simulink model "try_nelin2"  (R2014b)
settings: Solver=ode45  StartTime=0.0  StopTime=10.0  RelTol=1e-3
values from neighbouring files (symbols this model uses):
  d = 39.73e-3    (= 0.03973)    [liniarizare_crazyflie.m]
  g = 9.81    [liniarizare_crazyflie.m]
  Ixx = 1.395e-05    [liniarizare_crazyflie.m]
  Iyy = 1.436e-05    [liniarizare_crazyflie.m]
  Izz = 2.173e-05    [liniarizare_crazyflie.m]
  m = 0.27    [liniarizare_crazyflie.m]
  Th_coef = 3.1582e-10    [liniarizare_crazyflie.m]
  To_coef = 7.9379e-12    [liniarizare_crazyflie.m]
settings Model: Creator=uidd7441  LastModifiedBy=uidd7441

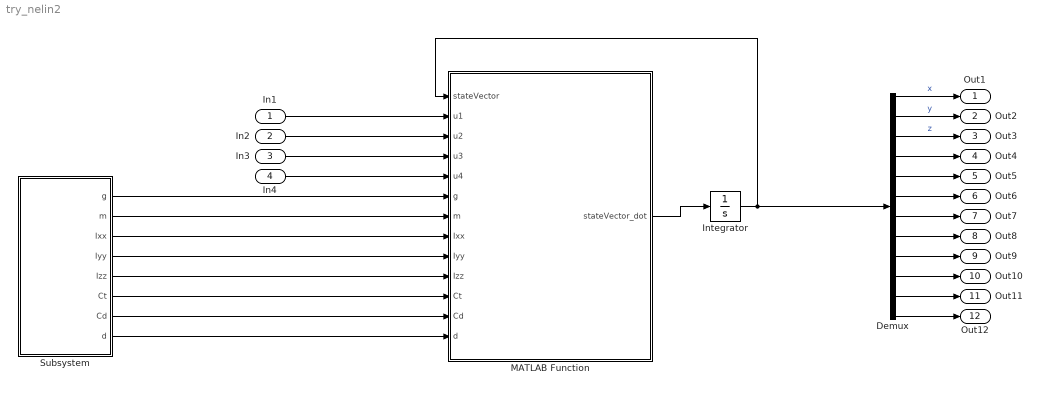
== system try_nelin2 ==
  In1 : Inport
  In2 : Inport  Port=2
  In3 : Inport  Port=3
  In4 : Inport  Port=4
  Demux : Demux  Outputs=12
  Integrator : Integrator  InitialCondition=[0 0 0 1 0 0 0 0 0 0 0 0]
  MATLAB Function : MATLAB Function  TreatAsAtomicUnit=on
  Subsystem : Subsystem
  Out1 : Outport
  Out2 : Outport  Port=2
  Out3 : Outport  Port=3
  Out4 : Outport  Port=4
  Out5 : Outport  Port=5
  Out6 : Outport  Port=6
  Out7 : Outport  Port=7
  Out8 : Outport  Port=8
  Out9 : Outport  Port=9
  Out10 : Outport  Port=10
  Out11 : Outport  Port=11
  Out12 : Outport  Port=12
  wires:
  Demux/5 -> Out5/1
  MATLAB Function/1(stateVector_dot) -> Integrator/1
  Integrator/1 -> Demux/1, MATLAB Function/1(stateVector)
  Demux/2 -> Out2/1  "y"
  Demux/4 -> Out4/1
  Demux/6 -> Out6/1
  Demux/3 -> Out3/1  "z"
  Demux/1 -> Out1/1  "x"
  Subsystem/4(Iyy) -> MATLAB Function/9(Iyy)
  Subsystem/7(Cd) -> MATLAB Function/12(Cd)
  Subsystem/5(Izz) -> MATLAB Function/10(Izz)
  Subsystem/6(Ct) -> MATLAB Function/11(Ct)
  Subsystem/8(d) -> MATLAB Function/13(d)
  Subsystem/1(g) -> MATLAB Function/6(g)
  Subsystem/2(m) -> MATLAB Function/7(m)
  Subsystem/3(Ixx) -> MATLAB Function/8(Ixx)
  Demux/9 -> Out9/1
  Demux/11 -> Out11/1
  Demux/10 -> Out10/1
  Demux/7 -> Out7/1
  Demux/8 -> Out8/1
  Demux/12 -> Out12/1
  In1/1 -> MATLAB Function/2(u1)
  In3/1 -> MATLAB Function/4(u3)
  In2/1 -> MATLAB Function/3(u2)
  In4/1 -> MATLAB Function/5(u4)

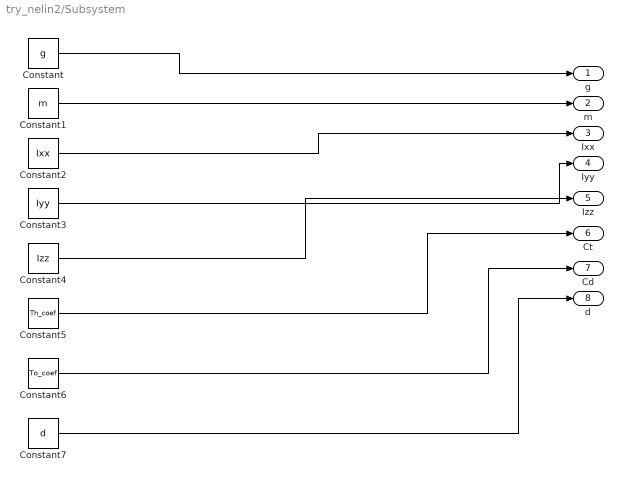
== system try_nelin2/Subsystem ==
  Constant : Constant  Value=g
  Constant1 : Constant  Value=m
  Constant2 : Constant  Value=Ixx
  Constant3 : Constant  Value=Iyy
  Constant4 : Constant  Value=Izz
  Constant5 : Constant  Value=Th_coef
  Constant6 : Constant  Value=To_coef
  Constant7 : Constant  Value=d
  g : Outport
  m : Outport  Port=2
  Ixx : Outport  Port=3
  Iyy : Outport  Port=4
  Izz : Outport  Port=5
  Ct : Outport  Port=6
  Cd : Outport  Port=7
  d : Outport  Port=8
  wires:
  Constant/1 -> g/1
  Constant5/1 -> Ct/1
  Constant4/1 -> Izz/1
  Constant7/1 -> d/1
  Constant2/1 -> Ixx/1
  Constant3/1 -> Iyy/1
  Constant1/1 -> m/1
  Constant6/1 -> Cd/1

== matlab function try_nelin2/MATLAB Function ==
  data: stateVector input; stateVector_dot output; u1 input; u2 input; u3 input; u4 input; g input; m input; Ixx input; Iyy input; Izz input; Ct input; Cd input; d input
function stateVector_dot = NeliniarModel(stateVector,u1,u2,u3,u4,g,m,Ixx,Iyy,Izz,Ct,Cd,d)
    
    %dx = [x y z yaw pitch roll x_rate y_rate z_rate yaw_rate pitch_rate
                %roll_rate]
    stateVector_dot = zeros(size(stateVector));
    
    Rot_InertialToBody = [cos(stateVector(5))*cos(stateVector(4)) cos(stateVector(5))*sin(stateVector(4)) -sin(stateVector(5)); ...
        sin(stateVector(6))*sin(stateVector(5))*cos(stateVector(4)) - cos(stateVector(6))*sin(stateVector(4))...
        sin(stateVector(6))*sin(stateVector(5))*sin(stateVector(4)) + cos(stateVector(6))*cos(stateVector(4))...
        sin(stateVector(6))*cos(stateVector(5)); ...
        cos(stateVector(6))*sin(stateVector(5))*cos(stateVector(4)) + sin(stateVector(6))*sin(stateVector(4))...
        cos(stateVector(6))*sin(stateVector(5))*sin(stateVector(4)) - sin(stateVector(6))*cos(stateVector(4))...
        cos(stateVector(6))*cos(stateVector(4))];
    
    stateVector_dot(1) = Rot_InertialToBody(1:3,1)'*[stateVector(7); stateVector(8); stateVector(9)];
    stateVector_dot(2) = Rot_InertialToBody(1:3,2)'*[stateVector(7); stateVector(8); stateVector(9)];
    stateVector_dot(3) = Rot_InertialToBody(1:3,3)'*[stateVector(7); stateVector(8); stateVector(9)];
    
    Rot_angles = [1 sin(stateVector(6))*tan(stateVector(5)) cos(stateVector(6))*tan(stateVector(5)); ...
        0 cos(stateVector(6)) -sin(stateVector(6)); ...
        0 sin(stateVector(6))/cos(stateVector(5)) cos(stateVector(6))/cos(stateVector(5))];
    
    stateVector_dot(6) = Rot_angles(1,1:3)*[stateVector(12); stateVector(11); stateVector(10)];
    stateVector_dot(5) = Rot_angles(2,1:3)*[stateVector(12); stateVector(11); stateVector(10)];
    stateVector_dot(4) = Rot_angles(3,1:3)*[stateVector(12); stateVector(11); stateVector(10)];
    
    % Ct = thrust coeff and Cd = aerodinamical drag
    Fz = Ct*(u1^2 + u2^2 + u3^2 + u4^2);
    
    cross_prod_rate = cross([stateVector(12); stateVector(11); stateVector(10)], [stateVector(7); stateVector(8); stateVector(10)]);
    second_termen = Rot_InertialToBody*[0;0;g];
    
    stateVector_dot(7) = - second_termen(1) - cross_prod_rate(1); 
    stateVector_dot(8) = - second_termen(2) - cross_prod_rate(2); 
    stateVector_dot(9) = Fz/m - second_termen(3) - cross_prod_rate(3); 
    
    Inertia_matrix = diag([Ixx Iyy Izz]);
    Mx = d*Ct/sqrt(2)*(-u1^2 - u2^2 + u3^2 + u4^2);
    My = d*Ct/sqrt(2)*(-u1^2 + u2^2 + u3^2 - u4^2);
    Mz = Cd*(-u1^2 + u2^2 - u3^2 + u4^2);
    
    Last_states = inv(Inertia_matrix)*([Mx; My; Mz] - cross([stateVector(12); stateVector(11); stateVector(10)], Inertia_matrix*[stateVector(12); stateVector(11); stateVector(10)]));
    stateVector_dot(10) = Last_states(3);
    stateVector_dot(11) = Last_states(2);
    stateVector_dot(12) = Last_states(1);
    
end
